simulink model "Add_Frame"  (R2013b)
settings: Solver=FixedStepDiscrete  StartTime=0.0  StopTime=200  RelTol=1e-3
InitFcn:
  | %% DSPBuilder Start
  | alt_dspbuilder_update_model(bdroot)
  | %% DSPBuilder End
StopFcn:
  | ed_out_script
undefined symbols (not defined in the file or in its folder): sigbuilder_block
libraries: allblocks_alteradspbuilder2 x118, simulink x5
(part 1 of 2)
settings Model: Creator=jb  LastModifiedBy=Given_Jiang

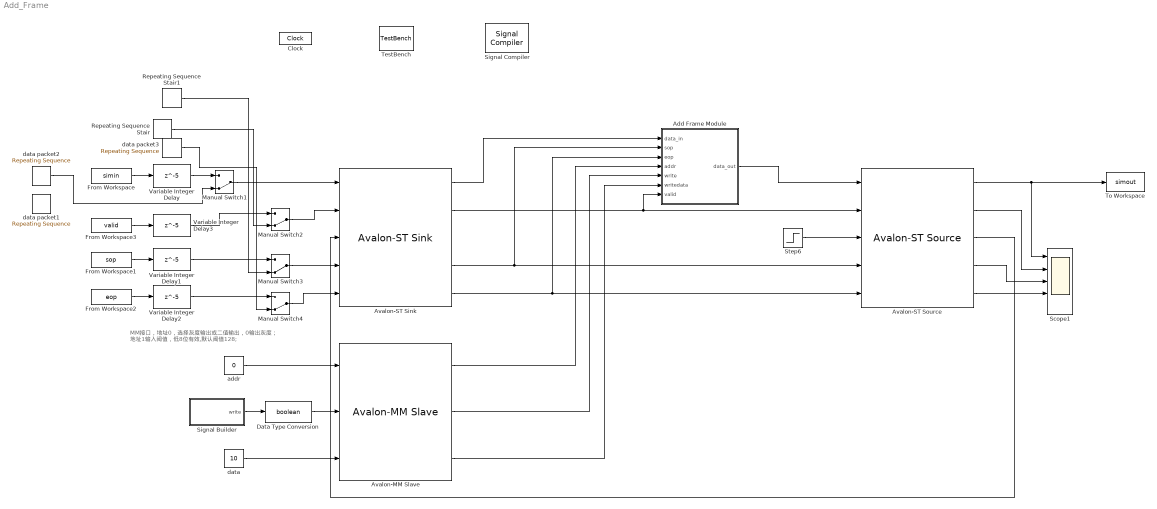
== system Add_Frame ==
  note: MM接口，地址0，选择灰度输出或二值输出，0输出灰度；
      |                  地址1输入阈值，低8位有效,默认阈值128;
  Add Frame Module : Subsystem
  Avalon-MM Slave : allblocks_alteradspbuilder2/Avalon-MM Slave  iofile=E:\FPGA\SOC\Quartus\quartus\dsp_builder\design\VIP_LIB\Add_Frame\tb_Add_Frame\Add%5FFrame_Avalon-MM+Slave_address.salt,E:\FPGA\SOC\Quartus\quartus\dsp_builder\design\VIP_LIB\Add_Frame\tb_Add_Frame\Add%5FFrame_Avalon-MM+Slave_write.salt,E:\FPGA\SOC\Quartus\quartus\dsp_builder\design\VIP_LIB\Add_Frame\tb_Add_Frame\Add%5FFrame_Avalon-MM+Slave_writedata.salt,  SpecifyClock=off  addrWidth=3  addrAlignment=Dynamic  addrType=Write  BusType=Unsigned Integer  bwl=32  bwr=0  byteEnable=off  flowCtrl=off  pipeline=off  waitStateFormat=Fixed  readWaitStateCycles=0  writeWaitStateCycles=1  readLatencyFormat=Fixed  readLatencyCycles=0  burst=off  maxBurst=4  irq=off  receiveBeginTransfer=off  useChipSelect=off  externalType=Inferred  PORTTYPE=Output
  Avalon-ST Sink : allblocks_alteradspbuilder2/Avalon-ST Sink  iofile=E:\FPGA\SOC\Quartus\quartus\dsp_builder\design\VIP_LIB\Add_Frame\tb_Add_Frame\Add%5FFrame_Avalon-ST+Sink_data.salt,E:\FPGA\SOC\Quartus\quartus\dsp_builder\design\VIP_LIB\Add_Frame\tb_Add_Frame\Add%5FFrame_Avalon-ST+Sink_valid.salt,E:\FPGA\SOC\Quartus\quartus\dsp_builder\design\VIP_LIB\Add_Frame\tb_Add_Frame\Add%5FFrame_Avalon-ST+Sink_ready.capture,E:\FPGA\SOC\Quartus\quartus\dsp_builder\design\VIP_LIB\Add_Frame\tb_Add_Frame\Add%5FFrame_Avalon-ST+Sink_startofpacket.salt,E:\FPGA\SOC\Quartus\quartus\dsp_builder\design\VIP_LIB\Add_Frame\tb_Add_Frame\Add%5FFrame_Avalon-ST+Sink_endofpacket.salt,  SpecifyClock=off  BusType=Unsigned Integer  bwl=24  bwr=0  symbolWidth=8  symbolsPerBeat=3  numOfChannels=0  numOfErrorDescriptors=0  endOfPacket=on  startOfPacket=on  empty=off  readyLatency=1  externalType=Inferred  PORTTYPE=Output
  Avalon-ST Source : allblocks_alteradspbuilder2/Avalon-ST Source  iofile=E:\FPGA\SOC\Quartus\quartus\dsp_builder\design\VIP_LIB\Add_Frame\tb_Add_Frame\Add%5FFrame_Avalon-ST+Source_data.capture,E:\FPGA\SOC\Quartus\quartus\dsp_builder\design\VIP_LIB\Add_Frame\tb_Add_Frame\Add%5FFrame_Avalon-ST+Source_valid.capture,E:\FPGA\SOC\Quartus\quartus\dsp_builder\design\VIP_LIB\Add_Frame\tb_Add_Frame\Add%5FFrame_Avalon-ST+Source_ready.salt,E:\FPGA\SOC\Quartus\quartus\dsp_builder\design\VIP_LIB\Add_Frame\tb_Add_Frame\Add%5FFrame_Avalon-ST+Source_startofpacket.capture,E:\FPGA\SOC\Quartus\quartus\dsp_builder\design\VIP_LIB\Add_Frame\tb_Add_Frame\Add%5FFrame_Avalon-ST+Source_endofpacket.capture,  SpecifyClock=off  BusType=Unsigned Integer  bwl=24  bwr=0  symbolWidth=8  symbolsPerBeat=3  numOfChannels=0  numOfErrorDescriptors=0  endOfPacket=on  startOfPacket=on  empty=off  readyLatency=1  externalType=Inferred  PORTTYPE=Input
  Clock : allblocks_alteradspbuilder2/Clock  ClockPeriod=7.5  ClockPeriodUnit=ns  SampleTime=1  ResetLatency=0  ResetRegisterCascadeDepth=0  SimulationStartCycle=5  PhaseOffset=0  Reset=aclr  ResetType=Active High  Export=off
  Data Type Conversion : DataTypeConversion  OutDataTypeStr=boolean
  From Workspace : FromWorkspace  VariableName=simin  Interpolate=off  OutputAfterFinalValue=Setting to zero
  From Workspace1 : FromWorkspace  VariableName=sop  Interpolate=off  OutputAfterFinalValue=Setting to zero
  From Workspace2 : FromWorkspace  VariableName=eop  Interpolate=off  OutputAfterFinalValue=Setting to zero
  From Workspace3 : FromWorkspace  VariableName=valid  Interpolate=off  OutputAfterFinalValue=Setting to zero
  Manual Switch{1..4} (4 alike) : ManualSwitch  CurrentSetting=0
  Repeating Sequence Stair : simulink/Sources/Repeating Sequence Stair  OutValues=[0 0 1 0 0 0 1 0 1].'  tsamp=-1  OutMin=[]  OutMax=[]  OutDataTypeStr=double  OutputDataTypeScalingMode=double  OutDataType=fixdt(0,8)  ConRadixGroup=Best Precision: Vector-wise  OutScaling=2^-12
  Repeating Sequence Stair1 : simulink/Sources/Repeating Sequence Stair  OutValues=[0 0 1 0 0 0 1 0 0 0].'  tsamp=-1  OutMin=[]  OutMax=[]  OutDataTypeStr=double  OutputDataTypeScalingMode=double  OutDataType=fixdt(0,8)  ConRadixGroup=Best Precision: Vector-wise  OutScaling=2^-12
  Scope1 : Scope  NumInputPorts=5
      settings: YMin=0~-5~-5~-5~-5  YMax=255~5~5~5~5  SampleTime=0.5
  Signal Builder : Subsystem  Tag=STV Subsys  LoadFcn=sigbuilder_block('load');  StartFcn=sigbuilder_block('start');  StopFcn=sigbuilder_block('stop');  ClipboardFcn=sigbuilder_block('clipboard');  mask(Sigbuilder block){}
      mask help: Simulink:masks:SigbuilderBlock_MD
      mask init:
      | if ~strcmp(get_param(bdroot(gcbh),'SimulationStatus'),'stopped') tuvar = sigbuilder_block('maskInit'); end
      settings: CopyFcn=sigbuilder_block('copy');  DeleteFcn=sigbuilder_block('delete');  ModelCloseFcn=sigbuilder_block('modelClose');  PreSaveFcn=sigbuilder_block('preSave');  PauseFcn=sigbuilder_block('pause');  ContinueFcn=sigbuilder_block('continue');  NameChangeFcn=sigbuilder_block('namechange');  OpenFcn=sigbuilder_block('open',[426 145.5 550.5 399.75 ]);  CloseFcn=sigbuilder_block('close');
      mask Display: plot(0, 0, 100, 100,[2, 2, 32, 32, 2], [68, 8, 8, 68, 68],[32, 2], [38, 38], [32, 19, 2],[53, 60, 44], [32, 17, 17, 2],[16, 16, 31, 31]);txt = getActiveGroup(gcbh);text(2, 100, txt,'verticalAlignment', 'top');
  Signal Compiler : allblocks_alteradspbuilder2/Signal Compiler  DeviceFamily=Cyclone V  DeviceName=AUTO  DisableEarlyHDLGeneration=off  EnableSignalTap=off  SignalTapDepth=128  UseBoardBlock=off  StpUseDefaultClock=on  StpClock=Clock  ExportDir=C:\Users\Given_Jiang\Documents
  Step6 : Step  SampleTime=0
  TestBench : allblocks_alteradspbuilder2/TestBench  enable=on  advancedMode=on  modelSimGui=on  maxDisplayErrors=10  mismatchErrorLevel=Error  simdatafile=E:\FPGA\SOC\Quartus\quartus\dsp_builder\design\VIP_LIB\Add_Frame\tb_Add_Frame\Add_Frame.simdata.tcl
  To Workspace : ToWorkspace  VariableName=simout  SampleTime=-1  SaveFormat=Structure With Time
  Variable Integer Delay{,1..3} (4 alike) : Delay  DelayLength=5
  addr : Constant  Value=0  OutDataTypeStr=uint8
  data : Constant  Value=10  OutDataTypeStr=uint32
  data packet1 : simulink/Sources/Repeating Sequence  rep_seq_t=[1 2 3 4 5 6 7 8 9 10 11]  rep_seq_y=uint32([0 0 15 524800 65536 14 0 1 2 3 0])
  data packet2 : simulink/Sources/Repeating Sequence  rep_seq_t=[1 2 3 4 5 6 7 8 9 10 11]  rep_seq_y=uint32([0 0 15 262400 0 15 0 0 0 0 0])
  data packet3 : simulink/Sources/Repeating Sequence  rep_seq_t=[1 2 3 4 5 6 7 8 9 10 11]  rep_seq_y=uint32([0 0 0 0 0 1 0 0 0 0 1])
  wires:
  Step6/1 -> Avalon-ST Source/3
  Avalon-ST Source/2 -> Scope1/2
  Avalon-ST Source/4 -> Scope1/3
  Avalon-ST Source/5 -> Scope1/4
  Avalon-ST Sink/2 -> Add Frame Module/7(valid), Avalon-ST Source/2
  Avalon-ST Source/3 -> Avalon-ST Sink/3
  Avalon-ST Sink/1 -> Add Frame Module/1(data_in)
  Avalon-ST Sink/4 -> Add Frame Module/2(sop), Avalon-ST Source/4
  Avalon-ST Sink/5 -> Add Frame Module/3(eop), Avalon-ST Source/5
  Avalon-MM Slave/1 -> Add Frame Module/4(addr)
  Avalon-MM Slave/2 -> Add Frame Module/5(write)
  Avalon-MM Slave/3 -> Add Frame Module/6(writedata)
  addr/1 -> Avalon-MM Slave/1
  data/1 -> Avalon-MM Slave/3
  Data Type Conversion/1 -> Avalon-MM Slave/2
  Signal Builder/1(write) -> Data Type Conversion/1
  Add Frame Module/1(data_out) -> Avalon-ST Source/1
  Variable Integer Delay1/1 -> Manual Switch3/1
  Variable Integer Delay2/1 -> Manual Switch4/1
  Variable Integer Delay3/1 -> Manual Switch2/1
  Manual Switch1/1 -> Avalon-ST Sink/1
  data packet2/1 -> Manual Switch1/2
  From Workspace/1 -> Variable Integer Delay/1
  Variable Integer Delay/1 -> Manual Switch1/1
  From Workspace1/1 -> Variable Integer Delay1/1
  From Workspace2/1 -> Variable Integer Delay2/1
  From Workspace3/1 -> Variable Integer Delay3/1
  Avalon-ST Source/1 -> To Workspace/1, Scope1/1
  Repeating Sequence Stair/1 -> Manual Switch2/2
  Manual Switch2/1 -> Avalon-ST Sink/2
  Repeating Sequence Stair1/1 -> Manual Switch3/2
  Manual Switch3/1 -> Avalon-ST Sink/4
  Manual Switch4/1 -> Avalon-ST Sink/5
  data packet3/1 -> Manual Switch4/2

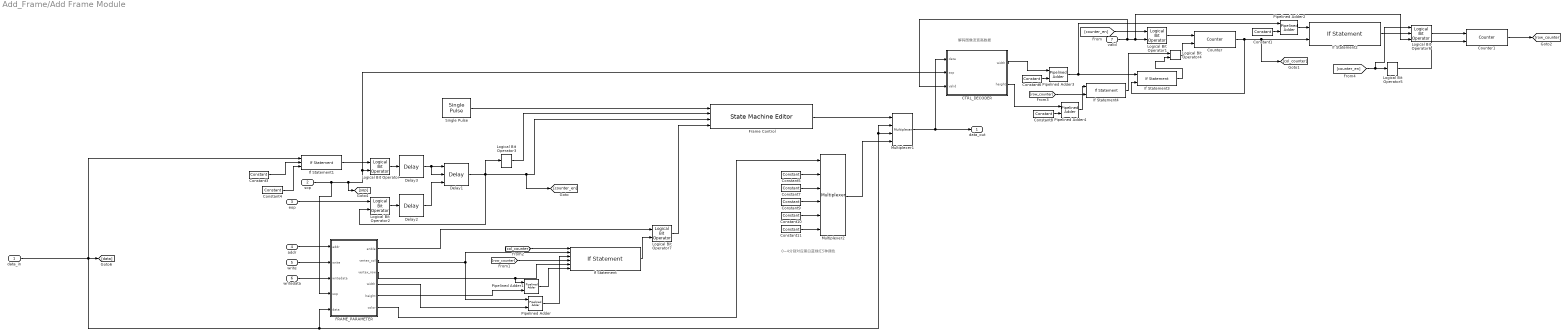
== system Add_Frame/Add Frame Module ==
  note: 解码图像流宽高数据
  note: 0~4分别对应黑白蓝绿红5种颜色
  data_in : Inport
  sop : Inport  Port=2
  eop : Inport  Port=3
  addr : Inport  Port=4
  write : Inport  Port=5
  writedata : Inport  Port=6
  valid : Inport  Port=7
  CTRL_DECODER : Subsystem
  Constant1 : allblocks_alteradspbuilder2/Constant  mask_cst=1  BusType=Unsigned Integer  bwl=16  bwr=0  roundMode=Truncate  satMode=Wrap  SpecifyClock=off  allowFloatingPointOverride=on  logOutputs=off  logFile=E:\FPGA\SOC\Quartus\quartus\dsp_builder\design\VIP_LIB\Add_Frame\tb_Add_Frame\Add%5FFrame_Add+Frame+Module_Constant1.fixedpointlog
  Constant10 : allblocks_alteradspbuilder2/Constant  mask_cst=65280  BusType=Unsigned Integer  bwl=24  bwr=0  roundMode=Truncate  satMode=Wrap  SpecifyClock=off  allowFloatingPointOverride=on  logOutputs=off  logFile=E:\FPGA\SOC\Quartus\quartus\dsp_builder\design\VIP_LIB\Add_Frame\tb_Add_Frame\Add%5FFrame_Add+Frame+Module_Constant10.fixedpointlog
  Constant11 : allblocks_alteradspbuilder2/Constant  mask_cst=16711680  BusType=Unsigned Integer  bwl=24  bwr=0  roundMode=Truncate  satMode=Wrap  SpecifyClock=off  allowFloatingPointOverride=on  logOutputs=off  logFile=E:\FPGA\SOC\Quartus\quartus\dsp_builder\design\VIP_LIB\Add_Frame\tb_Add_Frame\Add%5FFrame_Add+Frame+Module_Constant11.fixedpointlog
  Constant3 : allblocks_alteradspbuilder2/Constant  mask_cst=0  BusType=Unsigned Integer  bwl=24  bwr=0  roundMode=Truncate  satMode=Wrap  SpecifyClock=off  allowFloatingPointOverride=on  logOutputs=off  logFile=E:\FPGA\SOC\Quartus\quartus\dsp_builder\design\VIP_LIB\Add_Frame\tb_Add_Frame\Add%5FFrame_Add+Frame+Module_Constant3.fixedpointlog
  Constant4 : allblocks_alteradspbuilder2/Constant  mask_cst=15  BusType=Unsigned Integer  bwl=24  bwr=0  roundMode=Truncate  satMode=Wrap  SpecifyClock=off  allowFloatingPointOverride=on  logOutputs=off  logFile=E:\FPGA\SOC\Quartus\quartus\dsp_builder\design\VIP_LIB\Add_Frame\tb_Add_Frame\Add%5FFrame_Add+Frame+Module_Constant4.fixedpointlog
  Constant5 : allblocks_alteradspbuilder2/Constant  mask_cst=0  BusType=Unsigned Integer  bwl=24  bwr=0  roundMode=Truncate  satMode=Wrap  SpecifyClock=off  allowFloatingPointOverride=on  logOutputs=off  logFile=E:\FPGA\SOC\Quartus\quartus\dsp_builder\design\VIP_LIB\Add_Frame\tb_Add_Frame\Add%5FFrame_Add+Frame+Module_Constant5.fixedpointlog
  Constant6 : allblocks_alteradspbuilder2/Constant  mask_cst=1  BusType=Unsigned Integer  bwl=16  bwr=0  roundMode=Truncate  satMode=Wrap  SpecifyClock=off  allowFloatingPointOverride=on  logOutputs=off  logFile=E:\FPGA\SOC\Quartus\quartus\dsp_builder\design\VIP_LIB\Add_Frame\tb_Add_Frame\Add%5FFrame_Add+Frame+Module_Constant6.fixedpointlog
  Constant7 : allblocks_alteradspbuilder2/Constant  mask_cst=16777215  BusType=Unsigned Integer  bwl=24  bwr=0  roundMode=Truncate  satMode=Wrap  SpecifyClock=off  allowFloatingPointOverride=on  logOutputs=off  logFile=E:\FPGA\SOC\Quartus\quartus\dsp_builder\design\VIP_LIB\Add_Frame\tb_Add_Frame\Add%5FFrame_Add+Frame+Module_Constant7.fixedpointlog
  Constant8 : allblocks_alteradspbuilder2/Constant  mask_cst=1  BusType=Unsigned Integer  bwl=16  bwr=0  roundMode=Truncate  satMode=Wrap  SpecifyClock=off  allowFloatingPointOverride=on  logOutputs=off  logFile=E:\FPGA\SOC\Quartus\quartus\dsp_builder\design\VIP_LIB\Add_Frame\tb_Add_Frame\Add%5FFrame_Add+Frame+Module_Constant8.fixedpointlog
  Constant9 : allblocks_alteradspbuilder2/Constant  mask_cst=255  BusType=Unsigned Integer  bwl=24  bwr=0  roundMode=Truncate  satMode=Wrap  SpecifyClock=off  allowFloatingPointOverride=on  logOutputs=off  logFile=E:\FPGA\SOC\Quartus\quartus\dsp_builder\design\VIP_LIB\Add_Frame\tb_Add_Frame\Add%5FFrame_Add+Frame+Module_Constant9.fixedpointlog
  Counter : allblocks_alteradspbuilder2/Counter  BusType=Unsigned Integer  bwl=16  bwr=0  use_modulo=off  modulo=64  SpecifyClock=off  direction=Increment  use_sload=off  use_sset=off  svalue=1  use_clk_ena=off  use_ena=on  use_sclr=on  pipeline_display=1
  Counter1 : allblocks_alteradspbuilder2/Counter  BusType=Unsigned Integer  bwl=16  bwr=0  use_modulo=off  modulo=64  SpecifyClock=off  direction=Increment  use_sload=off  use_sset=off  svalue=1  use_clk_ena=off  use_ena=on  use_sclr=on  pipeline_display=1
  Delay1 : allblocks_alteradspbuilder2/Delay  pipeline=1  pipeline_display=1  ClockPhase=1  use_ena=on  use_sclr=on  allowFloatingPointOverride=on  logOutputs=off  logFile=E:\FPGA\SOC\Quartus\quartus\dsp_builder\design\VIP_LIB\Add_Frame\tb_Add_Frame\Add%5FFrame_Add+Frame+Module_Delay1.fixedpointlog  use_init=on  reset_value=0
  Delay2 : allblocks_alteradspbuilder2/Delay  pipeline=1  pipeline_display=1  ClockPhase=1  use_ena=off  use_sclr=off  allowFloatingPointOverride=on  logOutputs=off  logFile=E:\FPGA\SOC\Quartus\quartus\dsp_builder\design\VIP_LIB\Add_Frame\tb_Add_Frame\Add%5FFrame_Add+Frame+Module_Delay2.fixedpointlog  use_init=off  reset_value=0
  Delay3 : allblocks_alteradspbuilder2/Delay  pipeline=1  pipeline_display=1  ClockPhase=1  use_ena=off  use_sclr=off  allowFloatingPointOverride=on  logOutputs=off  logFile=E:\FPGA\SOC\Quartus\quartus\dsp_builder\design\VIP_LIB\Add_Frame\tb_Add_Frame\Add%5FFrame_Add+Frame+Module_Delay3.fixedpointlog  use_init=off  reset_value=0
  FRAME_PARAMETER : Subsystem
  Frame Control : allblocks_alteradspbuilder2/State Machine Editor  entityName=FrameControl_import  use_dynamic_feedthrough_data=on  inNames=reset ctrl_in data_in frame_in  inBwls=1 1 1 1  inBwrs="0  0  0  0"  inTypes=b b b b  inDelayed="0  1  1  1"  outNames=state  outBwls=3  outBwrs=0  outTypes=s  n_input_port=4  n_output_port=1  array_clocks=clock  xmlmapfile=E:\FPGA\SOC\Quartus\quartus\dsp_builder\lib\SimgenCMap.xml  vofile=DSPBuilder_Add_Frame_import\FrameControl.vo  use_systemC_model=off  is_megacore=off  smf_variation=|
      | /*                                                                         
      | WARNING: Do NOT edit the input and output ports in this file in a text     
      | editor if you plan to continue editing the block that represents it in     
      | the Block Editor! File corruption is VERY likely to occur.                 
      | Copyright (C) 1991-2013 Altera Corporation                                 
      | Your use of Altera Corporation's design tools, logic functions             
      | and other software and tools, and its AMPP partner logic                   
      | functions, and any output files from any of the foregoing                  
      | (including device programming or simulation files), and any                
      | associated documentation or information are expressly subject              
      | to the terms and conditions of the Altera Program License                  
      | Subscription Agreement, Altera MegaCore Function License                   
      | Agreement, or other applicable license agreement, including,               
      | without limitation, that your use is for the sole purpose of               
      | programming logic devices manufactured by Altera and sold by               
      | Altera or its authorized distributors.  Please refer to the                
      | applicable agreement for further details.                                  
      | Generated by Quartus II Version 13.1.0 Build 162 10/23/2013 SJ Full Version
      | Created on Sun Feb 22 16:00:25 2015                                        
      | */                                                                         
      | VERSION = "3.0";                                                           
      | HEADER                                                                     
      | (                                                                          
      | 	GENERAL{                                                                  
      | 		RMODE = "S";                                                             
      | 		RA_LEVEL = "H";                                                          
      | 		HOPT = "VHDL";                                                           
      | 	}                                                                         
      | 	SPORT{                                                                    
      | 		NAME = "clock";                                                          
      | 		PTYPE = "CI";                                                            
      | 		REG = "N";                                                               
      | 		OUTS = "N";                                                              
      | 	}                                                                         
      | 	SPORT{                                                                    
      | 		NAME = "reset";                                                          
      | 		PTYPE = "RI";                                                            
      | 		REG = "N";                                                               
      | 		OUTS = "N";                                                              
      | 	}                                                                         
      | 	SPORT{                                                                    
      | 		NAME = "ctrl_in";                                                        
      | 		PTYPE = "OI";                                                            
      | 		REG = "N";                                                               
      | 		OUTS = "N";                                                              
      | 	}                                                                         
      | 	SPORT{                                                                    
      | 		NAME = "data_in";                                                        
      | 		PTYPE = "OI";                                                            
      | 		REG = "N";                                                               
      | 		OUTS = "N";                                                              
      | 	}                                                                         
      | 	SPORT{                                                                    
      | 		NAME = "frame_in";                                                       
      | 		PTYPE = "OI";                                                            
      | 		REG = "N";                                                               
      | 		OUTS = "N";                                                              
      | 	}                                                                         
      | 	SPORT{                                                                    
      | 		NAME = "state[2:0]";                                                     
      | 		PTYPE = "OU";                                                            
      | 		REG = "N";                                                               
      | 		OUTS = "C";                                                              
      | 	}                                                                         
      | 	STATE{                                                                    
      | 		NAME = "IDLE";                                                           
      | 		STYPE = "RE";                                                            
      | 		PT = (296,296);                                                          
      | 		OUTP = "state[2:0]";                                                     
      | 		OUT_VALUE = "0";                                                         
      | 		COND = "";                                                               
      | 	}                                                                         
      | 	STATE{                                                                    
      | 		NAME = "DATA";                                                           
      | 		STYPE = "NR";                                                            
      | 		PT = (560,216);                                                          
      | 		OUTP = "state[2:0]";                                                     
      | 		OUT_VALUE = "2";                                                         
      | 		COND = "";                                                               
      | 	}                                                                         
      | 	STATE{                                                                    
      | 		NAME = "FRAME";                                                          
      | 		STYPE = "NR";                                                            
      | 		PT = (560,360);                                                          
      | 		OUTP = "state[2:0]";                                                     
      | 		OUT_VALUE = "4";                                                         
      | 		COND = "";                                                               
      | 	}                                                                         
      | 	STATE{                                                                    
      | 		NAME = "CTRL";                                                           
      | 		STYPE = "NR";                                                            
      | 		PT = (432,296);                                                          
      | 		OUTP = "state[2:0]";                                                     
      | 		OUT_VALUE = "1";                                                         
      | 		COND = "";                                                               
      | 	}                                                                         
      | 	TRANS{                                                                    
      | 		SSTATE = "IDLE";                                                         
      | 		DSTATE = "CTRL";                                                         
      | 		EQ = "ctrl_in==1";                                                       
      | 		PT = (345,320);                                                          
      | 		PT = (373,320);                                                          
      | 		PT = (402,320);                                                          
      | 		PT = (431,320);                                                          
      | 		PT = (387,330);                                                          
      | 	}                                                                         
      | 	TRANS{                                                                    
      | 		SSTATE = "FRAME";                                                        
      | 		DSTATE = "CTRL";                                                         
      | 		EQ = "(ctrl_in==1)&(data_in==0)&(frame_in==0)";                          
      | 		PT = (560,393);                                                          
      | 		PT = (530,376);                                                          
      | 		PT = (500,359);                                                          
      | 		PT = (469,341);                                                          
      | 		PT = (533,378);                                                          
      | 	}                                                                         
      | 	TRANS{                                                                    
      | 		SSTATE = "CTRL";                                                         
      | 		DSTATE = "DATA";                                                         
      | 		EQ = "(data_in==1)&(frame_in==0)";                                       
      | 		PT = (477,307);                                                          
      | 		PT = (509,293);                                                          
      | 		PT = (541,278);                                                          
      | 		PT = (574,263);                                                          
      | 		PT = (506,294);                                                          
      | 	}                                                                         
      | 	TRANS{                                                                    
      | 		SSTATE = "DATA";                                                         
      | 		DSTATE = "CTRL";                                                         
      | 		EQ = "(ctrl_in==1)&(frame_in==0)";                                       
      | 		PT = (574,263);                                                          
      | 		PT = (539,288);                                                          
      | 		PT = (503,315);                                                          
      | 		PT = (467,342);                                                          
      | 		PT = (542,286);                                                          
      | 	}                                                                         
      | 	TRANS{                                                                    
      | 		SSTATE = "CTRL";                                                         
      | 		DSTATE = "FRAME";                                                        
      | 		EQ = "(data_in==0)&(frame_in==1)";                                       
      | 		PT = (480,321);                                                          
      | 		PT = (507,338);                                                          
      | 		PT = (534,355);                                                          
      | 		PT = (562,373);                                                          
      | 		PT = (504,336);                                                          
      | 	}                                                                         
      | 	TRANS{                                                                    
      | 		SSTATE = "DATA";                                                         
      | 		DSTATE = "FRAME";                                                        
      | 		EQ = "(ctrl_in==0)&(frame_in==1)";                                       
      | 		PT = (584,265);                                                          
      | 		PT = (584,296);                                                          
      | 		PT = (584,327);                                                          
      | 		PT = (584,359);                                                          
      | 		PT = (594,311);                                                          
      | 	}                                                                         
      | 	TRANS{                                                                    
      | 		SSTATE = "FRAME";                                                        
      | 		DSTATE = "DATA";                                                         
      | 		EQ = "(ctrl_in==0)&(data_in==1)&(frame_in==0)";                          
      | 		PT = (604,369);                                                          
      | 		PT = (604,331);                                                          
      | 		PT = (604,293);                                                          
      | 		PT = (604,255);                                                          
      | 		PT = (614,312);                                                          
      | 	}                                                                         
      | )                                                                          
      | END
  If Statement : allblocks_alteradspbuilder2/If Statement  user_inputs=6  if_expression=(((a>b)|(a=b))&((a<c)|(a=c))&(d=e))|((d>e)&(d<f)&(a=b))|((d>e)&(d<f)&(a=c))|(((a>b)|(a=b))&((a<c)|(a=c))&(d=f))  BusType=Unsigned Integer  bwl=16  bwr=0  pipeline_display=1  use_else_output=off  use_elseif_input=off
  If Statement1 : allblocks_alteradspbuilder2/If Statement  user_inputs=3  if_expression=(a=b)&(a~c)  BusType=Unsigned Integer  bwl=24  bwr=0  pipeline_display=1  use_else_output=off  use_elseif_input=off
  If Statement2 : allblocks_alteradspbuilder2/If Statement  user_inputs=2  if_expression=(a=b)  BusType=Unsigned Integer  bwl=16  bwr=0  pipeline_display=1  use_else_output=off  use_elseif_input=off
  If Statement3 : allblocks_alteradspbuilder2/If Statement  user_inputs=2  if_expression=(a=b)  BusType=Unsigned Integer  bwl=16  bwr=0  pipeline_display=1  use_else_output=off  use_elseif_input=off
  If Statement4 : allblocks_alteradspbuilder2/If Statement  user_inputs=2  if_expression=(a=b)  BusType=Unsigned Integer  bwl=16  bwr=0  pipeline_display=1  use_else_output=off  use_elseif_input=off
  Logical Bit Operator{,1..2,7} (4 alike) : allblocks_alteradspbuilder2/Logical Bit Operator  LogicalOperator=AND  user_inputs=2  pipeline_display=0
  Logical Bit Operator3 : allblocks_alteradspbuilder2/Logical Bit Operator  LogicalOperator=NOT  user_inputs=2  pipeline_display=0
  Logical Bit Operator4 : allblocks_alteradspbuilder2/Logical Bit Operator  LogicalOperator=OR  user_inputs=2  pipeline_display=0
  Logical Bit Operator5 : allblocks_alteradspbuilder2/Logical Bit Operator  LogicalOperator=NOT  user_inputs=2  pipeline_display=0
  Logical Bit Operator6 : allblocks_alteradspbuilder2/Logical Bit Operator  LogicalOperator=AND  user_inputs=3  pipeline_display=0
  Multiplexer1 : allblocks_alteradspbuilder2/Multiplexer  numInputs=3  pipeline=0  oneHot=on  pipeline_display=0  use_ena=off  use_aclr=off  allowFloatingPointOverride=on  logOutputs=off  logFile=E:\FPGA\SOC\Quartus\quartus\dsp_builder\design\VIP_LIB\Add_Frame\tb_Add_Frame\Add%5FFrame_Add+Frame+Module_Multiplexer1.fixedpointlog
  Multiplexer2 : allblocks_alteradspbuilder2/Multiplexer  numInputs=5  pipeline=0  oneHot=off  pipeline_display=0  use_ena=off  use_aclr=off  allowFloatingPointOverride=on  logOutputs=off  logFile=E:\FPGA\SOC\Quartus\quartus\dsp_builder\design\VIP_LIB\Add_Frame\tb_Add_Frame\Add%5FFrame_Add+Frame+Module_Multiplexer2.fixedpointlog
  Pipelined Adder : allblocks_alteradspbuilder2/Pipelined Adder  BusType=Unsigned Integer  bwl=16  bwr=0  pipeline=0  pipeline_display=0  AddSubDirection=ADD  use_cin=off  use_ovl=off  use_addsub=off  use_ena=off  use_aclr=off  or_aclr_inputs=on
  Pipelined Adder1 : allblocks_alteradspbuilder2/Pipelined Adder  BusType=Unsigned Integer  bwl=16  bwr=0  pipeline=0  pipeline_display=0  AddSubDirection=ADD  use_cin=off  use_ovl=off  use_addsub=off  use_ena=off  use_aclr=off  or_aclr_inputs=on
  Pipelined Adder2 : allblocks_alteradspbuilder2/Pipelined Adder  BusType=Unsigned Integer  bwl=16  bwr=0  pipeline=0  pipeline_display=0  AddSubDirection=SUB  use_cin=off  use_ovl=off  use_addsub=off  use_ena=off  use_aclr=off  or_aclr_inputs=on
  Pipelined Adder3 : allblocks_alteradspbuilder2/Pipelined Adder  BusType=Unsigned Integer  bwl=16  bwr=0  pipeline=0  pipeline_display=0  AddSubDirection=SUB  use_cin=off  use_ovl=off  use_addsub=off  use_ena=off  use_aclr=off  or_aclr_inputs=on
  Pipelined Adder4 : allblocks_alteradspbuilder2/Pipelined Adder  BusType=Unsigned Integer  bwl=16  bwr=0  pipeline=0  pipeline_display=0  AddSubDirection=SUB  use_cin=off  use_ovl=off  use_addsub=off  use_ena=off  use_aclr=off  or_aclr_inputs=on
  Single Pulse : allblocks_alteradspbuilder2/Single Pulse  signal_type=Step Down  impulse_width=1  delay=1  SpecifyClock=off  use_ena=off  use_sclr=off
  data_out : Outport
  wires:
  If Statement1/1 -> Logical Bit Operator/1
  Delay1/1 -> [counter_en], Frame Control/3, Logical Bit Operator2/2, Logical Bit Operator3/1
  Constant3/1 -> If Statement1/2
  Constant4/1 -> If Statement1/3
  eop/1 -> Logical Bit Operator2/1
  Logical Bit Operator2/1 -> Delay2/1
  Delay2/1 -> Delay1/3
  data_in/1 -> [data], FRAME_PARAMETER/5(data), Multiplexer1/3, Multiplexer1/2, If Statement1/1
  Logical Bit Operator/1 -> Delay3/1
  Delay3/1 -> Delay1/2, Delay1/1
  FRAME_PARAMETER/2(vertex_col) -> If Statement/2, Pipelined Adder/1
  addr/1 -> FRAME_PARAMETER/1(addr)
  write/1 -> FRAME_PARAMETER/2(write)
  writedata/1 -> FRAME_PARAMETER/3(writedata)
  FRAME_PARAMETER/4(width) -> Pipelined Adder/2
  Pipelined Adder/1 -> If Statement/3
  Single Pulse/1 -> Frame Control/1
  Logical Bit Operator7/1 -> Frame Control/4
  Multiplexer1/1 -> CTRL_DECODER/1(data), data_out/1
  Frame Control/1 -> Multiplexer1/1
  Multiplexer2/1 -> Multiplexer1/4
  FRAME_PARAMETER/3(vertex_row) -> Pipelined Adder1/1, If Statement/5
  [row_counter] -> If Statement/4
  [col_counter] -> If Statement/1
  FRAME_PARAMETER/5(height) -> Pipelined Adder1/2
  Pipelined Adder1/1 -> If Statement/6
  Logical Bit Operator3/1 -> Frame Control/2
  sop/1 -> FRAME_PARAMETER/4(sop), [sop], CTRL_DECODER/2(sop), Logical Bit Operator/2
  Counter/1 -> If Statement3/2, [col_counter], If Statement2/2
  Counter1/1 -> [row_counter]
  [counter_en] -> Logical Bit Operator1/1
  valid/1 -> CTRL_DECODER/3(valid), Logical Bit Operator6/3, Logical Bit Operator1/2
  Logical Bit Operator1/1 -> Counter/1
  Pipelined Adder3/1 -> Pipelined Adder2/1, If Statement3/1
  If Statement3/1 -> Logical Bit Operator4/2
  Pipelined Adder2/1 -> If Statement2/1
  Constant1/1 -> Pipelined Adder2/2
  Constant6/1 -> Pipelined Adder3/2
  CTRL_DECODER/1(width) -> Pipelined Adder3/1
  Logical Bit Operator4/1 -> Counter/2
  If Statement4/1 -> Logical Bit Operator4/1
  Logical Bit Operator5/1 -> Counter1/2
  [row_counter] -> If Statement4/2
  [counter_en] -> Logical Bit Operator6/1, Logical Bit Operator5/1
  Logical Bit Operator6/1 -> Counter1/1
  If Statement2/1 -> Logical Bit Operator6/2
  CTRL_DECODER/2(height) -> Pipelined Adder4/1
  Constant8/1 -> Pipelined Adder4/2
  Pipelined Adder4/1 -> If Statement4/1
  FRAME_PARAMETER/1(enble) -> Logical Bit Operator7/1
  If Statement/1 -> Logical Bit Operator7/2
  FRAME_PARAMETER/6(color) -> Multiplexer2/1
  Constant5/1 -> Multiplexer2/2
  Constant7/1 -> Multiplexer2/3
  Constant9/1 -> Multiplexer2/4
  Constant10/1 -> Multiplexer2/5
  Constant11/1 -> Multiplexer2/6

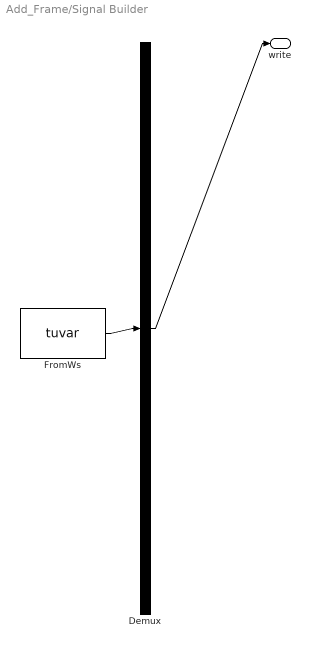
== system Add_Frame/Signal Builder ==
  Demux : Demux  Tag=STV Demux  Outputs=1
  FromWs : FromWorkspace  Tag=STV FromWs  VariableName=tuvar  SampleTime=0  OutputAfterFinalValue=Setting to zero
      SigBuilderData=|
      | common.afterFinalStr = 'Set to zero'
      | common.sampleTime = '0'
      | dataSet.timeRange = [0 10]
      | dataSet.name = 'Group 1'
      | sbobj.Groups.Name = 'Group 1'
      | sbobj.Groups.Signals.Name = 'write'
      | sbobj.Groups.Signals.XData = [0 3 3 5 5 10]
      | sbobj.Groups.Signals.YData = [0 0 0.995 1 0 0]
  write : Outport  Tag=STV Outport
  wires:
  Demux/1 -> write/1
  FromWs/1 -> Demux/1

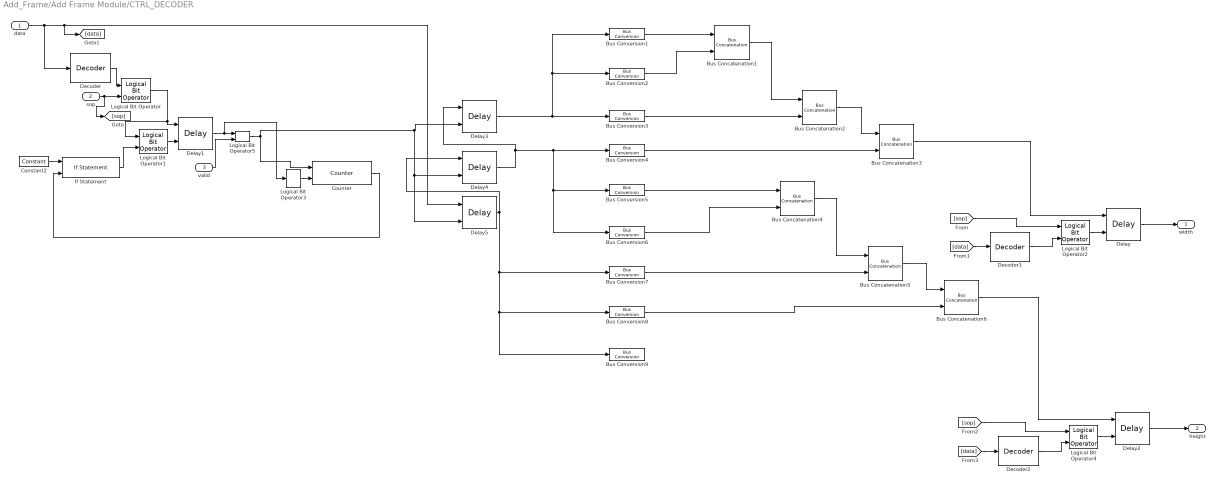
== system Add_Frame/Add Frame Module/CTRL_DECODER ==
  data : Inport
  sop : Inport  Port=2
  valid : Inport  Port=3
  Bus Concatenation1 : allblocks_alteradspbuilder2/Bus Concatenation  isSigned=off  awidth=4  bwidth=4  pipeline_display=0
  Bus Concatenation2 : allblocks_alteradspbuilder2/Bus Concatenation  isSigned=off  awidth=8  bwidth=4  pipeline_display=0
  Bus Concatenation3 : allblocks_alteradspbuilder2/Bus Concatenation  isSigned=off  awidth=12  bwidth=4  pipeline_display=0
  Bus Concatenation4 : allblocks_alteradspbuilder2/Bus Concatenation  isSigned=off  awidth=4  bwidth=4  pipeline_display=0
  Bus Concatenation5 : allblocks_alteradspbuilder2/Bus Concatenation  isSigned=off  awidth=8  bwidth=4  pipeline_display=0
  Bus Concatenation6 : allblocks_alteradspbuilder2/Bus Concatenation  isSigned=off  awidth=12  bwidth=4  pipeline_display=0
  Bus Conversion1 : allblocks_alteradspbuilder2/Bus Conversion  BusType=Unsigned Integer  ibwl=24  ibwr=1  bwl=4  bwr=1  bitToConnectToOutputLSB=0  round=off  saturate=off  pipeline_display=0
  Bus Conversion2 : allblocks_alteradspbuilder2/Bus Conversion  BusType=Unsigned Integer  ibwl=24  ibwr=1  bwl=4  bwr=1  bitToConnectToOutputLSB=8  round=off  saturate=off  pipeline_display=0
  Bus Conversion3 : allblocks_alteradspbuilder2/Bus Conversion  BusType=Unsigned Integer  ibwl=24  ibwr=1  bwl=4  bwr=1  bitToConnectToOutputLSB=16  round=off  saturate=off  pipeline_display=0
  Bus Conversion4 : allblocks_alteradspbuilder2/Bus Conversion  BusType=Unsigned Integer  ibwl=24  ibwr=1  bwl=4  bwr=1  bitToConnectToOutputLSB=0  round=off  saturate=off  pipeline_display=0
  Bus Conversion5 : allblocks_alteradspbuilder2/Bus Conversion  BusType=Unsigned Integer  ibwl=24  ibwr=1  bwl=4  bwr=1  bitToConnectToOutputLSB=8  round=off  saturate=off  pipeline_display=0
  Bus Conversion6 : allblocks_alteradspbuilder2/Bus Conversion  BusType=Unsigned Integer  ibwl=24  ibwr=1  bwl=4  bwr=1  bitToConnectToOutputLSB=16  round=off  saturate=off  pipeline_display=0
  Bus Conversion7 : allblocks_alteradspbuilder2/Bus Conversion  BusType=Unsigned Integer  ibwl=24  ibwr=1  bwl=4  bwr=1  bitToConnectToOutputLSB=0  round=off  saturate=off  pipeline_display=0
  Bus Conversion8 : allblocks_alteradspbuilder2/Bus Conversion  BusType=Unsigned Integer  ibwl=24  ibwr=1  bwl=4  bwr=1  bitToConnectToOutputLSB=8  round=off  saturate=off  pipeline_display=0
  Bus Conversion9 : allblocks_alteradspbuilder2/Bus Conversion  BusType=Unsigned Integer  ibwl=24  ibwr=1  bwl=4  bwr=1  bitToConnectToOutputLSB=16  round=off  saturate=off  pipeline_display=0
  Constant2 : allblocks_alteradspbuilder2/Constant  mask_cst=2  BusType=Unsigned Integer  bwl=3  bwr=0  roundMode=Truncate  satMode=Wrap  SpecifyClock=off  allowFloatingPointOverride=on  logOutputs=off  logFile=E:\FPGA\SOC\Quartus\quartus\dsp_builder\design\VIP_LIB\Add_Frame\tb_Add_Frame\Add%5FFrame_Add+Frame+Module_CTRL%5FDECODER_Constant2.fixedpointlog
  Counter : allblocks_alteradspbuilder2/Counter  BusType=Unsigned Integer  bwl=3  bwr=0  use_modulo=off  modulo=5  SpecifyClock=off  direction=Increment  use_sload=off  use_sset=off  svalue=1  use_clk_ena=off  use_ena=on  use_sclr=on  pipeline_display=1
  Decoder : allblocks_alteradspbuilder2/Decoder  BusType=Unsigned Integer  bwl=24  bwr=2  registered=off  pipeline_display=0  value=15
  Decoder1 : allblocks_alteradspbuilder2/Decoder  BusType=Unsigned Integer  bwl=24  bwr=2  registered=off  pipeline_display=0  value=0
  Decoder2 : allblocks_alteradspbuilder2/Decoder  BusType=Unsigned Integer  bwl=24  bwr=2  registered=off  pipeline_display=0  value=0
  Delay : allblocks_alteradspbuilder2/Delay  pipeline=1  pipeline_display=1  ClockPhase=1  use_ena=on  use_sclr=off  allowFloatingPointOverride=on  logOutputs=off  logFile=E:\FPGA\SOC\Quartus\quartus\dsp_builder\design\VIP_LIB\Add_Frame\tb_Add_Frame\Add%5FFrame_Add+Frame+Module_CTRL%5FDECODER_Delay.fixedpointlog  use_init=on  reset_value=0
  Delay1 : allblocks_alteradspbuilder2/Delay  pipeline=1  pipeline_display=1  ClockPhase=1  use_ena=on  use_sclr=off  allowFloatingPointOverride=on  logOutputs=off  logFile=E:\FPGA\SOC\Quartus\quartus\dsp_builder\design\VIP_LIB\Add_Frame\tb_Add_Frame\Add%5FFrame_Add+Frame+Module_CTRL%5FDECODER_Delay1.fixedpointlog  use_init=off  reset_value=1
  Delay2 : allblocks_alteradspbuilder2/Delay  pipeline=1  pipeline_display=1  ClockPhase=1  use_ena=on  use_sclr=off  allowFloatingPointOverride=on  logOutputs=off  logFile=E:\FPGA\SOC\Quartus\quartus\dsp_builder\design\VIP_LIB\Add_Frame\tb_Add_Frame\Add%5FFrame_Add+Frame+Module_CTRL%5FDECODER_Delay2.fixedpointlog  use_init=on  reset_value=0
  Delay3 : allblocks_alteradspbuilder2/Delay  pipeline=1  pipeline_display=1  ClockPhase=1  use_ena=on  use_sclr=off  allowFloatingPointOverride=on  logOutputs=off  logFile=E:\FPGA\SOC\Quartus\quartus\dsp_builder\design\VIP_LIB\Add_Frame\tb_Add_Frame\Add%5FFrame_Add+Frame+Module_CTRL%5FDECODER_Delay3.fixedpointlog  use_init=off  reset_value=1
  Delay4 : allblocks_alteradspbuilder2/Delay  pipeline=1  pipeline_display=1  ClockPhase=1  use_ena=on  use_sclr=off  allowFloatingPointOverride=on  logOutputs=off  logFile=E:\FPGA\SOC\Quartus\quartus\dsp_builder\design\VIP_LIB\Add_Frame\tb_Add_Frame\Add%5FFrame_Add+Frame+Module_CTRL%5FDECODER_Delay4.fixedpointlog  use_init=off  reset_value=1
  Delay5 : allblocks_alteradspbuilder2/Delay  pipeline=1  pipeline_display=1  ClockPhase=1  use_ena=on  use_sclr=off  allowFloatingPointOverride=on  logOutputs=off  logFile=E:\FPGA\SOC\Quartus\quartus\dsp_builder\design\VIP_LIB\Add_Frame\tb_Add_Frame\Add%5FFrame_Add+Frame+Module_CTRL%5FDECODER_Delay5.fixedpointlog  use_init=off  reset_value=1
  If Statement : allblocks_alteradspbuilder2/If Statement  user_inputs=2  if_expression=(a<b)  BusType=Inferred  bwl=8  bwr=0  pipeline_display=1  use_else_output=off  use_elseif_input=off
  Logical Bit Operator{,2,4..5} (4 alike) : allblocks_alteradspbuilder2/Logical Bit Operator  LogicalOperator=AND  user_inputs=2  pipeline_display=0
  Logical Bit Operator1 : allblocks_alteradspbuilder2/Logical Bit Operator  LogicalOperator=OR  user_inputs=2  pipeline_display=0
  Logical Bit Operator3 : allblocks_alteradspbuilder2/Logical Bit Operator  LogicalOperator=NOT  user_inputs=2  pipeline_display=0
  width : Outport
  height : Outport  Port=2
  wires:
  data/1 -> Decoder/1, [data], Delay5/1
  Delay4/1 -> Bus Conversion6/1, Bus Conversion5/1, Bus Conversion4/1, Delay3/1
  Delay5/1 -> Bus Conversion9/1, Bus Conversion8/1, Bus Conversion7/1, Delay4/1
  Bus Concatenation3/1 -> Delay/1
  Logical Bit Operator5/1 -> Delay5/2, Delay4/2, Delay3/2, Counter/1
  Decoder/1 -> Logical Bit Operator/1
  sop/1 -> [sop], Logical Bit Operator/2
  Logical Bit Operator/1 -> Delay1/1, Logical Bit Operator1/1
  Counter/1 -> If Statement/2
  Constant2/1 -> If Statement/1
  If Statement/1 -> Logical Bit Operator1/2
  Logical Bit Operator1/1 -> Delay1/2
  Logical Bit Operator3/1 -> Counter/2
  [sop] -> Logical Bit Operator2/1
  [data] -> Decoder1/1
  Decoder1/1 -> Logical Bit Operator2/2
  Logical Bit Operator2/1 -> Delay/2
  Delay/1 -> width/1
  Bus Concatenation6/1 -> Delay2/1
  [sop] -> Logical Bit Operator4/1
  [data] -> Decoder2/1
  Decoder2/1 -> Logical Bit Operator4/2
  Logical Bit Operator4/1 -> Delay2/2
  Delay2/1 -> height/1
  Delay3/1 -> Bus Conversion3/1, Bus Conversion2/1, Bus Conversion1/1
  Bus Conversion1/1 -> Bus Concatenation1/1
  Bus Conversion2/1 -> Bus Concatenation1/2
  Bus Concatenation1/1 -> Bus Concatenation2/1
  Bus Conversion3/1 -> Bus Concatenation2/2
  Bus Conversion4/1 -> Bus Concatenation3/2
  Bus Concatenation2/1 -> Bus Concatenation3/1
  Bus Concatenation4/1 -> Bus Concatenation5/1
  Bus Conversion7/1 -> Bus Concatenation5/2
  Bus Conversion8/1 -> Bus Concatenation6/2
  Bus Concatenation5/1 -> Bus Concatenation6/1
  Bus Conversion5/1 -> Bus Concatenation4/1
  Bus Conversion6/1 -> Bus Concatenation4/2
  Delay1/1 -> Logical Bit Operator3/1, Logical Bit Operator5/1
  valid/1 -> Logical Bit Operator5/2
